simulink model "Retificador_nao_controlado"  (R2017a)
settings: Solver=VariableStepAuto  StartTime=0.0  StopTime=1/30  RelTol=1e-3
libraries: fl_lib x14, nesl_utility x8
settings Model: Creator=gabriel  LastModifiedBy=gabriel

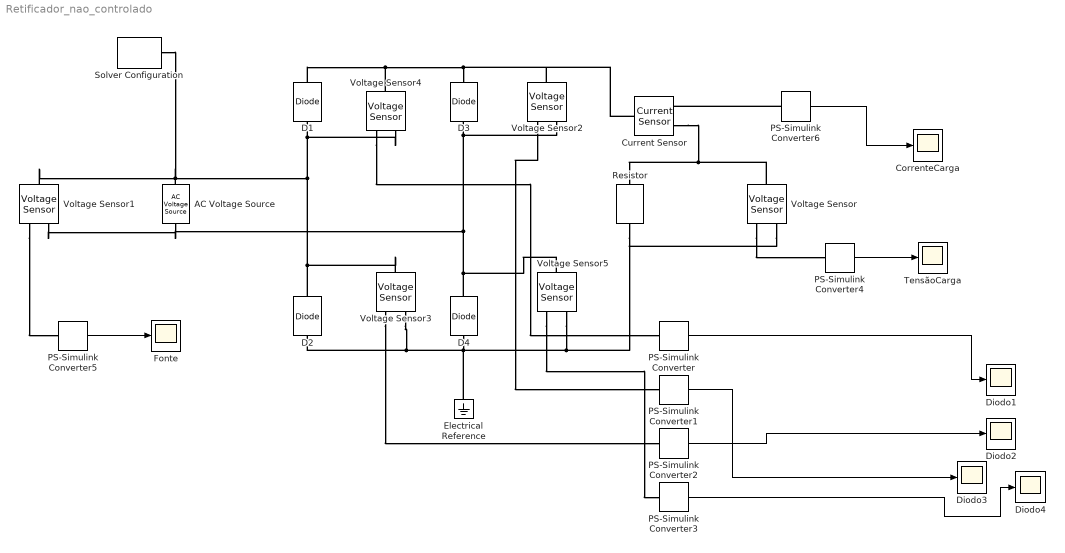
== system Retificador_nao_controlado ==
  AC Voltage Source : fl_lib/Electrical/Electrical Sources/AC Voltage Source  amp=130*sqrt(2) V  shift=0 deg  frequency=60 Hz  omega=0 rad/s
  CorrenteCarga : Scope
  Current Sensor : fl_lib/Electrical/Electrical Sensors/Current Sensor
  "D1 " : fl_lib/Electrical/Electrical Elements/Diode  Vf=0.6 V  Ron=0.3 Ohm  Goff=1e-8 1/Ohm  i_specify=off  i_priority=None  i=0 A  i_nominal_specify=off  i_nominal_unit=A  i_nominal_value=1  v_specify=off  v_priority=None  v=0 V  v_nominal_specify=off  v_nominal_unit=V  v_nominal_value=1
  D2 : fl_lib/Electrical/Electrical Elements/Diode  Vf=0.6 V  Ron=0.3 Ohm  Goff=1e-8 1/Ohm  i_specify=off  i_priority=None  i=0 A  i_nominal_specify=off  i_nominal_unit=A  i_nominal_value=1  v_specify=off  v_priority=None  v=0 V  v_nominal_specify=off  v_nominal_unit=V  v_nominal_value=1
  D3 : fl_lib/Electrical/Electrical Elements/Diode  Vf=0.6 V  Ron=0.3 Ohm  Goff=1e-8 1/Ohm  i_specify=off  i_priority=None  i=0 A  i_nominal_specify=off  i_nominal_unit=A  i_nominal_value=1  v_specify=off  v_priority=None  v=0 V  v_nominal_specify=off  v_nominal_unit=V  v_nominal_value=1
  D4 : fl_lib/Electrical/Electrical Elements/Diode  Vf=0.6 V  Ron=0.3 Ohm  Goff=1e-8 1/Ohm  i_specify=off  i_priority=None  i=0 A  i_nominal_specify=off  i_nominal_unit=A  i_nominal_value=1  v_specify=off  v_priority=None  v=0 V  v_nominal_specify=off  v_nominal_unit=V  v_nominal_value=1
  Diodo{1..4} (4 alike) : Scope
  Electrical Reference : fl_lib/Electrical/Electrical Elements/Electrical Reference
  Fonte : Scope
  PS-Simulink Converter{,1..6} (7 alike) : nesl_utility/PS-Simulink Converter  PhysicalDomain=network_engine_domain  SubClassName=ps_output  LeftPortType=input  RightPortType=output  PseudoPeriodic=off  Frequencies=[]  Unit=1  AffineConversion=off
  Resistor : fl_lib/Electrical/Electrical Elements/Resistor  R=66.5 Ohm  i_specify=off  i_priority=None  i=0 A  i_nominal_specify=off  i_nominal_unit=A  i_nominal_value=1  v_specify=off  v_priority=None  v=0 V  v_nominal_specify=off  v_nominal_unit=V  v_nominal_value=1
  Solver Configuration : nesl_utility/Solver Configuration  PhysicalDomain=network_engine_domain  SubClassName=solver  LeftPortType=input  RightPortType=generic  Accelerate=off  Tones=[]  Harmonics=[]  SimulateNoise=off  Profile=off  UseLocalSampling=off  EnableSwitchedLinearOptims=on  FrequencyDomain=off  UseCCode=off  RelTol=0.001  AbsTol=1e-06  MinStep=1e-09  ToWorkspace=off  RevertToSquareIcSolve=off  NumHomotopyIterations=100  PhasorMode=off  PhasorModeNumHarmonics=1  OverrideAbsTol=off  DoDC=off  ResidualTolerance=1e-09  UseLocalSolver=off  LocalSolverChoice=NE_BACKWARD_EULER_ADVANCER  LocalSolverSampleTime=0.001  DoFixedCost=off  MaxNonlinIter=3  MaxModeIter=2  LinearAlgebra=Sparse  DelaysMemoryBudget=1024  AutomaticFiltering=on  FilteringTimeConstant=0.001
  TensãoCarga : Scope
  Voltage Sensor{,1..5} (6 alike) : fl_lib/Electrical/Electrical Sensors/Voltage Sensor
  wires:
  PS-Simulink Converter/1 -> Diodo1/1
  PS-Simulink Converter2/1 -> Diodo2/1
  PS-Simulink Converter3/1 -> Diodo4/1
  PS-Simulink Converter4/1 -> TensãoCarga/1
  PS-Simulink Converter5/1 -> Fonte/1
  PS-Simulink Converter1/1 -> Diodo3/1
  PS-Simulink Converter6/1 -> CorrenteCarga/1
  connections:
  D2/RConn1 -- Voltage Sensor3/LConn1 -- Solver Configuration/RConn1 -- AC Voltage Source/LConn1 -- Voltage Sensor1/LConn1 -- Voltage Sensor4/RConn2 -- "D1 "/LConn1
  D4/RConn1 -- Voltage Sensor5/LConn1 -- Voltage Sensor1/RConn2 -- AC Voltage Source/RConn1 -- Voltage Sensor2/RConn2 -- D3/LConn1
  D4/LConn1 -- Voltage Sensor5/RConn2 -- Resistor/RConn1 -- Voltage Sensor/RConn2 -- Electrical Reference/LConn1 -- Voltage Sensor3/RConn2 -- D2/LConn1
  "D1 "/RConn1 -- Voltage Sensor4/LConn1 -- Current Sensor/LConn1 -- Voltage Sensor2/LConn1 -- D3/RConn1
  Voltage Sensor4/RConn1 -- PS-Simulink Converter/LConn1
  Voltage Sensor2/RConn1 -- PS-Simulink Converter1/LConn1
  Voltage Sensor3/RConn1 -- PS-Simulink Converter2/LConn1
  Voltage Sensor5/RConn1 -- PS-Simulink Converter3/LConn1
  Voltage Sensor/RConn1 -- PS-Simulink Converter4/LConn1
  Voltage Sensor1/RConn1 -- PS-Simulink Converter5/LConn1
  Voltage Sensor/LConn1 -- Current Sensor/RConn2 -- Resistor/LConn1
  PS-Simulink Converter6/LConn1 -- Current Sensor/RConn1
